simulink model "LightControl_Harness"  (R2018a)
settings: Solver=VariableStepAuto  StartTime=0.0  StopTime=10.0  RelTol=1e-3
undefined symbols (not defined in the file): sigbuilder_block
settings Model: Creator=jonathancoulter  LastModifiedBy=jonathancoulter

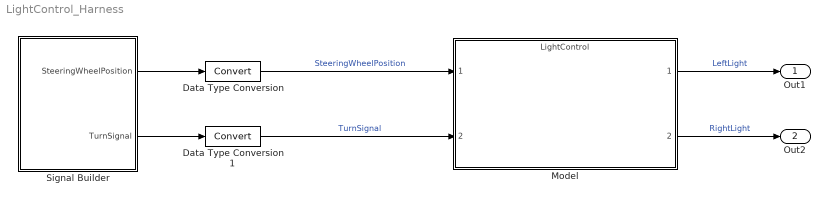
== system LightControl_Harness ==
  Data Type Conversion : DataTypeConversion
  Data Type Conversion1 : DataTypeConversion
  Model : ModelReference  ModelNameDialog=LightControl.slx  ModelReferenceVersion=1.16
  Signal Builder : Subsystem  Tag=STV Subsys  LoadFcn=sigbuilder_block('load');  StartFcn=sigbuilder_block('start');  StopFcn=sigbuilder_block('stop');  ClipboardFcn=sigbuilder_block('clipboard');  mask(Sigbuilder block){tuvar=[0:10]}
      mask help: Simulink:masks:SigbuilderBlock_MD
      mask init:
      | if ~strcmp(get_param(bdroot(gcbh),'SimulationStatus'),'stopped') tuvar = sigbuilder_block('maskInit'); end
      settings: CopyFcn=sigbuilder_block('copy');  DeleteFcn=sigbuilder_block('delete');  ModelCloseFcn=sigbuilder_block('modelClose');  PreSaveFcn=sigbuilder_block('preSave');  PauseFcn=sigbuilder_block('pause');  ContinueFcn=sigbuilder_block('continue');  NameChangeFcn=sigbuilder_block('namechange');  OpenFcn=sigbuilder_block('open',[437.6 199.2 550.4 400 ]);  CloseFcn=sigbuilder_block('close');
      mask Display: plot(0, 0, 100, 100,[2, 2, 32, 32, 2], [68, 8, 8, 68, 68],[32, 2], [38, 38], [32, 19, 2],[53, 60, 44], [32, 17, 17, 2],[16, 16, 31, 31]);txt = getActiveGroup(gcbh);text(2, 100, txt,'verticalAlignment', 'top');
  Out1 : Outport
  Out2 : Outport  Port=2
  wires:
  Signal Builder/1(SteeringWheelPosition) -> Data Type Conversion/1
  Signal Builder/2(TurnSignal) -> Data Type Conversion1/1
  Model/1 -> Out1/1  "LeftLight"
  Data Type Conversion/1 -> Model/1  "SteeringWheelPosition"
  Data Type Conversion1/1 -> Model/2  "TurnSignal"
  Model/2 -> Out2/1  "RightLight"

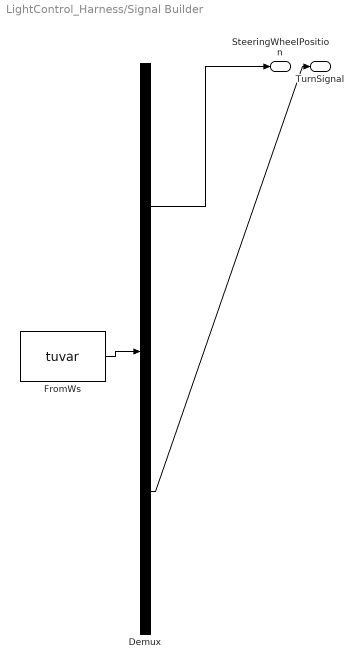
== system LightControl_Harness/Signal Builder ==
  Demux : Demux  Tag=STV Demux  Outputs=2
  FromWs : FromWorkspace  Tag=STV FromWs  VariableName=tuvar  SampleTime=0
      SigBuilderData=|
      | common.afterFinalStr = 'Extrapolate'
      | common.sampleTime = 0
      | dataSet.timeRange = [0 10]
      | dataSet.name = 'Group 1'
      | sbobj.Groups.Name = 'Group 1'
      | sbobj.Groups.Signals(1).Name = 'SteeringWheelPosition'
      | sbobj.Groups.Signals(1).XData = [0 2.5 5 7.5 10]
      | sbobj.Groups.Signals(1).YData = [0 25 -25 25 0]
      | sbobj.Groups.Signals(2).Name = 'TurnSignal'
      | sbobj.Groups.Signals(2).XData = [0 10]
      | sbobj.Groups.Signals(2).YData = [0 0]
  SteeringWheelPosition : Outport  Tag=STV Outport
  TurnSignal : Outport  Tag=STV Outport  Port=2
  wires:
  Demux/1 -> SteeringWheelPosition/1
  FromWs/1 -> Demux/1
  Demux/2 -> TurnSignal/1
